simulink model "sldemo_mdladv"  (Simulink 7.6)
settings: Solver=VariableStepDiscrete  StartTime=0.0  StopTime=10.0  RelTol=1e-3
Description:
  | Model Advisor
  | 
  | This demonstration shows the capabilities of the Model Advisor to check
  | a model or subsystem for conditions and configuration settings that can
  | result in inaccurate or inefficient simulation of the system represented
  | by the model or generation of inefficient code from the model. The Model
  | Advisor produces a report that lists all the suboptimal conditions or
  | settings that it finds, suggesting better model configuration settings where
  | appropriate.
  | 
  | The Model Advisor can started through menus or the command line and
  | can also be configured and used through a comprehensive API.
settings Model: Creator=The MathWorks Inc.  CovMetricSettings=d  ExtModeTrigMode=oneshot  ExtModeArmWhenConnect=off  ExtModeAutoUpdateStatusClock=off
settings DataIOCC: LimitDataPoints=off  SaveOutput=off  SaveTime=off
settings OptimizationCC: BlockReduction=off  BooleanDataType=off  InlineInvariantSignals=on  InitFltsAndDblsToZero=on  EfficientMapNaN2IntZero=off  BufferReusableBoundary=off
settings DebuggingCC: SaveWithParameterizedLinksMsg=none  SignalResolutionControl=TryResolveAllWithWarning  SolverPrmCheckMsg=none  MultiTaskDSMMsg=warning  MultiTaskCondExecSysMsg=none  SigSpecEnsureSampleTimeMsg=none  IntegerOverflowMsg=none  UnconnectedInputMsg=none  UnconnectedOutputMsg=none  BusObjectLabelMismatch=none
settings RTWCC: IncludeERTFirstTime=on
settings GRTTargetCC: TargetFcnLib=ansi_tfl_tmw.mat

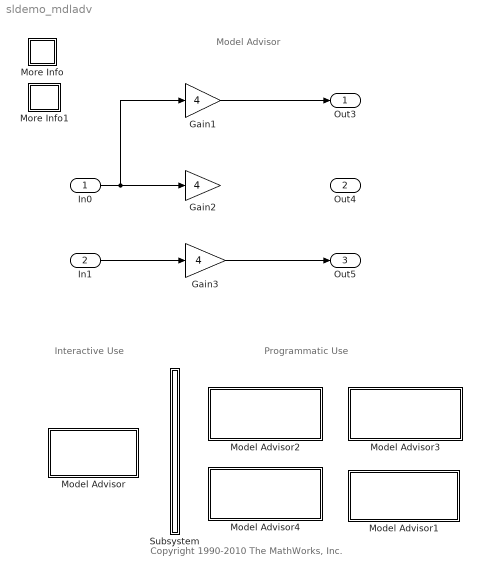
== system sldemo_mdladv ==
  note: Model Advisor
  note: Copyright 1990-2010 The MathWorks, Inc.
  note: Interactive Use
  note: Programmatic Use
  In0 : Inport  OutDataTypeStr=uint8  Interpolate=off
  In1 : Inport  Port=2  OutDataTypeStr=uint8  Interpolate=off
  Gain1 : Gain  Gain=4  OutDataTypeStr=Inherit: Same as input  ParamDataTypeStr=Inherit: Same as input
  Gain2 : Gain  Gain=4  ParamDataTypeStr=fixdt(1,32,0)  SaturateOnIntegerOverflow=on  OutDataTypeStr=Inherit: Same as input
  Gain3 : Gain  Gain=4  ParamDataTypeStr=fixdt(1,32,0)  OutDataTypeStr=Inherit: Same as input
  Model Advisor : Subsystem  mask{attrib_overrides={}}
      mask prompts: attrib_overrides "List of attributes to preserve (cell of strings):"
      mask help: Enter the attributes of the configuration set that you want preserved. Otherwise, the default configuration script will override your current settings.
      settings: OpenFcn=modeladvisor(bdroot);
      mask Display:
      | text(.05,.5,['Launch Model\n',...
      | 	  'Advisor ..','.'])
  Model Advisor1 : Subsystem  mask{attrib_overrides={}}
      mask prompts: attrib_overrides "List of attributes to preserve (cell of strings):"
      mask help: Enter the attributes of the configuration set that you want preserved. Otherwise, the default configuration script will override your current settings.
      settings: OpenFcn=edit sldemo_mdladv_helper;
      mask Display:
      | text(.05,.5,['View demo\n',...
      | 	  'source code'])
  Model Advisor2 : Subsystem  mask{attrib_overrides={}}
      mask prompts: attrib_overrides "List of attributes to preserve (cell of strings):"
      mask help: Enter the attributes of the configuration set that you want preserved. Otherwise, the default configuration script will override your current settings.
      settings: OpenFcn=sldemo_mdladv_helper('selectCheckAll')
      mask Display: text(.05,.5,['Select all checks \n and run'])
  Model Advisor3 : Subsystem  mask{attrib_overrides={}}
      mask prompts: attrib_overrides "List of attributes to preserve (cell of strings):"
      mask help: Enter the attributes of the configuration set that you want preserved. Otherwise, the default configuration script will override your current settings.
      settings: OpenFcn=sldemo_mdladv_helper('selectTaskAll')
      mask Display: text(.05,.5,['Select all tasks \n and run'])
  Model Advisor4 : Subsystem  mask{attrib_overrides={}}
      mask prompts: attrib_overrides "List of attributes to preserve (cell of strings):"
      mask help: Enter the attributes of the configuration set that you want preserved. Otherwise, the default configuration script will override your current settings.
      settings: OpenFcn=sldemo_mdladv_helper('ShowCheckPassFail')
      mask Display: text(.05,.5,['View collected \n result status'])
  More Info : Subsystem
      settings: OpenFcn=showdemo('sldemo_mdladv');
      mask Display: disp('?')
  More Info1 : Subsystem
      settings: OpenFcn=helpview([docroot '/mapfiles/simulink.map'], 'model_advisor');
      mask Display: disp('Doc')
  Subsystem : Subsystem
  Out3 : Outport
  Out4 : Outport  Port=2
  Out5 : Outport  Port=3
  wires:
  Gain1/1 -> Out3/1
  Gain3/1 -> Out5/1
  In0/1 -> Gain1/1, Gain2/1
  In1/1 -> Gain3/1

== system sldemo_mdladv/Model Advisor ==

== system sldemo_mdladv/Model Advisor1 ==

== system sldemo_mdladv/Model Advisor2 ==

== system sldemo_mdladv/Model Advisor3 ==

== system sldemo_mdladv/Model Advisor4 ==

== system sldemo_mdladv/More Info ==

== system sldemo_mdladv/More Info1 ==

== system sldemo_mdladv/Subsystem ==
